simulink model "nms_3Dmodel_inv_wAnkleCPG"  (R2016b)
settings: Solver=ode3  StartTime=0.0  StopTime=tend  FixedStep=ts  RelTol=1e-3  EnableMultiTasking=on
InitFcn:
  | runScripts_inv;
values from neighbouring files (symbols this model uses):
  c = 0.05    [IID_nms_MechInit.m]    (also in nms_MechInit.m)
  c_jointstop = 0.3 / (pi/180)    (= 17.1887338539)    [IID_nms_MechInit.m]    (also in nms_MechInit.m)
  CPG_On = 1    [setCPGPar.m]    (also in setCPGPar_inv.m)
  CtrlPar_FP = [alpha0 alpha_cd alpha_cv]    [setCtrlPar.m]
  CtrlPar_FP_R = [R_hipR0 R_hipR_cd R_hipR_cv]    [setCtrlPar.m]
  CtrlPar_LL = l_clr    [setCtrlPar.m]
  CtrlPar_St = [StPreStim St_M1 St_M2 St_M3 St_M4 St_M5 St_M11]    [setCtrlPar.m]
  CtrlPar_St_R = [R_StPreStim R_St_M1 R_St_M3 R_St_M4]    [setCtrlPar.m]
  CtrlPar_Sw = [SwPreStim SwPhasePari SwPhaseParii SwCtrlPar_H SwCtrlPar_A      SwCtrlPar_Ki SwCtrlPar_Kii SwCtrlPar_Kiii SwCtrlPar_StP]    [setCtrlPar.m]
  CtrlPar_Sw_R = [R_SwPreStim R_Sw_M6]    [setCtrlPar.m]
  CtrlPar_theta0 = parBlCtrl(1)      *1*pi/180    [setCtrlPar.m]
  CtrlPar_Tr = [Tr_St_sup Tr_Sw]    [setCtrlPar.m]
  CtrlPar_Tr_R = [R_Tr_St_sup R_Tr_Sw]    [setCtrlPar.m]
  eref = 0.04    [IID_nms_MechInit.m]    (also in nms_MechInit.m)
  FmaxBFSH = 350    [nms_MechInit.m]
  FmaxGAS = 1500    [IID_nms_MechInit.m]    (also in nms_MechInit.m)
  FmaxGLU = 1500    [IID_nms_MechInit.m]    (also in nms_MechInit.m)
  FmaxHAB = 3000    [nms_MechInit.m]
  FmaxHAD = 4500    [nms_MechInit.m]
  FmaxHAM = 3000    [IID_nms_MechInit.m]    (also in nms_MechInit.m)
  FmaxHFL = 2000    [IID_nms_MechInit.m]    (also in nms_MechInit.m)
  FmaxRF = 1200    [nms_MechInit.m]
  FmaxSOL = 4000    [IID_nms_MechInit.m]    (also in nms_MechInit.m)
  FmaxTA = 800    [IID_nms_MechInit.m]    (also in nms_MechInit.m)
  FmaxVAS = 6000    [IID_nms_MechInit.m]    (also in nms_MechInit.m)
  init_a_tgt = 70*pi/180    (= 1.2217304764)    [setInitPar.m]
  init_a_tgtR = 90*pi/180    (= 1.57079632679)    [setInitPar.m]
  K = 5    [IID_nms_MechInit.m]    (also in nms_MechInit.m)
  leg_l = [D12_T D12_S]    [nms_MechInit.m]
  LongDelay = 0.020    (= 0.02)    [IID_setCtrlPar.m]    (also in nms_MechInit.m = 0.01)
  LongLoopDelay = 0.030    (= 0.03)    [nms_MechInit.m]
  loptBFSH = 0.12    [nms_MechInit.m]
  loptGAS = 0.05    [IID_nms_MechInit.m]    (also in nms_MechInit.m)
  loptGLU = 0.11    [IID_nms_MechInit.m]    (also in nms_MechInit.m)
  loptHAB = 0.09    [nms_MechInit.m]
  loptHAD = 0.10    (= 0.1)    [nms_MechInit.m]
  loptHAM = 0.10    (= 0.1)    [IID_nms_MechInit.m]    (also in nms_MechInit.m)
  loptHFL = 0.11    [IID_nms_MechInit.m]    (also in nms_MechInit.m)
  loptRF = 0.08    [nms_MechInit.m]
  loptSOL = 0.04    [IID_nms_MechInit.m]    (also in nms_MechInit.m)
  loptTA = 0.06    [IID_nms_MechInit.m]    (also in nms_MechInit.m)
  loptVAS = 0.08    [IID_nms_MechInit.m]    (also in nms_MechInit.m)
  lslackBFSH = 0.10    (= 0.1)    [nms_MechInit.m]
  lslackGAS = 0.40    (= 0.4)    [IID_nms_MechInit.m]    (also in nms_MechInit.m)
  lslackGLU = 0.13    [IID_nms_MechInit.m]    (also in nms_MechInit.m)
  lslackHAB = 0.07    [nms_MechInit.m]
  lslackHAD = 0.18    [nms_MechInit.m]
  lslackHAM = 0.31    [IID_nms_MechInit.m]    (also in nms_MechInit.m)
  lslackHFL = 0.10    (= 0.1)    [IID_nms_MechInit.m]    (also in nms_MechInit.m)
  lslackRF = 0.35    [nms_MechInit.m]
  lslackSOL = 0.26    [IID_nms_MechInit.m]    (also in nms_MechInit.m)
  lslackTA = 0.24    [IID_nms_MechInit.m]    (also in nms_MechInit.m)
  lslackVAS = 0.23    [IID_nms_MechInit.m]    (also in nms_MechInit.m)
  massBFSH = 2    [nms_MechInit.m]
  massGAS = 0.45    [IID_nms_MechInit.m]    (also in nms_MechInit.m)
  massGLU = 1.4    [IID_nms_MechInit.m]    (also in nms_MechInit.m)
  massHAB = 1.145    [nms_MechInit.m]
  massHAD = 1.91    [nms_MechInit.m]
  massHAM = 1.82    [IID_nms_MechInit.m]    (also in nms_MechInit.m)
  massHFL = 1.87    [IID_nms_MechInit.m]    (also in nms_MechInit.m)
  massRF = 1    [nms_MechInit.m]
  massSOL = 1.36    [IID_nms_MechInit.m]    (also in nms_MechInit.m)
  massTA = 0.29    [IID_nms_MechInit.m]    (also in nms_MechInit.m)
  massVAS = 2.91    [IID_nms_MechInit.m]    (also in nms_MechInit.m)
  MidDelay = 0.010    (= 0.01)    [IID_setCtrlPar.m]    (also in nms_MechInit.m = 0.005)
  N = 1.5    [IID_nms_MechInit.m]    (also in cmaes_parfor.m = size(x,1); nms_MechInit.m)
  phi12_LowLimit = 70*pi/180    (= 1.2217304764)    [IID_nms_MechInit.m]    (also in nms_MechInit.m)
  phi12_UpLimit = 130*pi/180    (= 2.26892802759)    [IID_nms_MechInit.m]    (also in nms_MechInit.m)
  phi23_UpLimit = 175*pi/180    (= 3.05432619099)    [IID_nms_MechInit.m]    (also in nms_MechInit.m)
  phi34_UpLimit = 230*pi/180    (= 4.01425727959)    [IID_nms_MechInit.m]    (also in nms_MechInit.m)
  phi34R_LowLimit = -15*pi/180    (= -0.261799387799)    [nms_MechInit.m]
  phi34R_UpLimit = 50*pi/180    (= 0.872664625997)    [nms_MechInit.m]
  phimaxGASa = 110*pi/180    (= 1.91986217719)    [IID_nms_MechInit.m]    (also in nms_MechInit.m = 1.74532925199)
  phimaxGASk = 140*pi/180    (= 2.44346095279)    [IID_nms_MechInit.m]    (also in nms_MechInit.m)
  phimaxRFk = 165*pi/180    (= 2.87979326579)    [nms_MechInit.m]
  phimaxSOL = 110*pi/180    (= 1.91986217719)    [IID_nms_MechInit.m]    (also in nms_MechInit.m = 1.74532925199)
  phimaxTA = 80*pi/180    (= 1.3962634016)    [IID_nms_MechInit.m]    (also in nms_MechInit.m)
  phimaxVAS = 165*pi/180    (= 2.87979326579)    [IID_nms_MechInit.m]    (also in nms_MechInit.m)
  phirefBFSH = 160*pi/180    (= 2.79252680319)    [nms_MechInit.m]
  phirefGASa = 80*pi/180    (= 1.3962634016)    [IID_nms_MechInit.m]    (also in nms_MechInit.m)
  phirefGASk = 165*pi/180    (= 2.87979326579)    [IID_nms_MechInit.m]    (also in nms_MechInit.m)
  phirefGLU = 150*pi/180    (= 2.61799387799)    [IID_nms_MechInit.m]    (also in nms_MechInit.m = 2.09439510239)
  phirefHAB = 10*pi/180    (= 0.174532925199)    [nms_MechInit.m]
  phirefHAD = 15*pi/180    (= 0.261799387799)    [nms_MechInit.m]
  phirefHAMh = 155*pi/180    (= 2.70526034059)    [IID_nms_MechInit.m]    (also in nms_MechInit.m = 2.61799387799)
  phirefHAMk = 180*pi/180    (= 3.14159265359)    [IID_nms_MechInit.m]    (also in nms_MechInit.m)
  phirefHFL = 180*pi/180    (= 3.14159265359)    [IID_nms_MechInit.m]    (also in nms_MechInit.m = 2.79252680319)
  phirefRFh = 170*pi/180    (= 2.96705972839)    [nms_MechInit.m]
  phirefRFk = 125*pi/180    (= 2.18166156499)    [nms_MechInit.m]
  phirefSOL = 80*pi/180    (= 1.3962634016)    [IID_nms_MechInit.m]    (also in nms_MechInit.m = 1.57079632679)
  phirefTA = 110*pi/180    (= 1.91986217719)    [IID_nms_MechInit.m]    (also in nms_MechInit.m)
  phirefVAS = 125*pi/180    (= 2.18166156499)    [IID_nms_MechInit.m]    (also in nms_MechInit.m = 2.09439510239)
  phiScaleGASa = acos(rGASamin/rGASamax)/(phiminGASa-phimaxGASa)    [nms_MechInit.m]
  phiScaleGASk = acos(rGASkmin/rGASkmax)/(phiminGASk-phimaxGASk)    [nms_MechInit.m]
  phiScaleRFk = acos(rRFkmin/rRFkmax)/(phiminRFk-phimaxRFk)    [nms_MechInit.m]
  phiScaleSOL = acos(rSOLmin/rSOLmax)/(phiminSOL-phimaxSOL)    [nms_MechInit.m]
  phiScaleTA = acos(rTAmin/rTAmax)/(phiminTA-phimaxTA)    [nms_MechInit.m]
  phiScaleVAS = acos(rVASmin/rVASmax)/(phiminVAS-phimaxVAS)    [nms_MechInit.m]
  rBFSH = 0.04    [nms_MechInit.m]
  rGASamax = 0.06    [nms_MechInit.m]
  rGASkmax = 0.05    [nms_MechInit.m]
  rGLU = 0.10    (= 0.1)    [IID_nms_MechInit.m]    (also in nms_MechInit.m = 0.08)
  rHAB = 0.06    [nms_MechInit.m]
  rHAD = 0.03    [nms_MechInit.m]
  rHAMh = 0.08    [IID_nms_MechInit.m]    (also in nms_MechInit.m)
  rHAMk = 0.05    [IID_nms_MechInit.m]    (also in nms_MechInit.m)
  rHFL = 0.10    (= 0.1)    [IID_nms_MechInit.m]    (also in nms_MechInit.m = 0.08)
  rhoBFSH = 0.7    [nms_MechInit.m]
  rhoGASa = 0.7    [IID_nms_MechInit.m]    (also in nms_MechInit.m)
  rhoGASk = 0.7    [IID_nms_MechInit.m]    (also in nms_MechInit.m)
  rhoGLU = 0.5    [IID_nms_MechInit.m]    (also in nms_MechInit.m)
  rhoHAB = 0.7    [nms_MechInit.m]
  rhoHAD = 1    [nms_MechInit.m]
  rhoHAMh = 0.7    [IID_nms_MechInit.m]    (also in nms_MechInit.m = 0.5)
  rhoHAMk = 0.7    [IID_nms_MechInit.m]    (also in nms_MechInit.m = 0.5)
  rhoHFL = 0.5    [IID_nms_MechInit.m]    (also in nms_MechInit.m)
  rhoRFh = 0.3    [nms_MechInit.m]
  rhoRFk = 0.5    [nms_MechInit.m]
  rhoSOL = 0.5    [IID_nms_MechInit.m]    (also in nms_MechInit.m)
  rhoTA = 0.7    [IID_nms_MechInit.m]    (also in nms_MechInit.m)
  ... (+55 more)
libraries: simulink_extras x30, nmc x30, simulink x22, NMCCPG_Library x13, powerlib_meascontrol x5
(part 12 of 12)

== system nms_3Dmodel_inv_wAnkleCPG/NMC Model/Neural Control Layer (Spinal Cord Control)/L Swing Phase (sagittal)/kneeii_damp and hold &kneeiii_leg stop &kneeiv_stance preparation ==
  note: Knee Phase i
  CtrlPar : Inport
  a_tgt : Inport  Port=2
  LceRF : Inport  Port=3
  LceHAM : Inport  Port=4
  VceHAM : Inport  Port=5
  VceVAS : Inport  Port=6
  VceBFSH : Inport  Port=7
  VceRF : Inport  Port=8
  LceHFL : Inport  Port=9
  LceGLU : Inport  Port=10
  LceVAS : Inport  Port=11
  Enable : EnablePort  StatesWhenEnabling=reset  ZeroCross=off
  Compare To Constant : simulink/Logic and Bit Operations/Compare To Constant  relop=<=  const=0  OutDataTypeStr=uint8  ZeroCross=off
  Constant1 : Constant  Value=0  OutDataTypeStr=boolean
  Constant2 : Constant  Value=0  OutDataTypeStr=boolean
  Constant3 : Constant  Value=0  OutDataTypeStr=boolean
  Constant4 : Constant
  Constant5 : Constant
  Demux1 : Demux  Outputs=5
  Divide1 : Product
  Divide2 : Product
  Logical Operator : Logic  Operator=NOT  AllPortsSameDT=off  OutDataTypeStr=boolean
  Logical Operator1 : Logic  AllPortsSameDT=off  OutDataTypeStr=boolean
  Relational Operator : RelationalOperator  Operator=<=  OutDataTypeStr=boolean  ZeroCross=off  RndMeth=Nearest
  Relational Operator1 : RelationalOperator  OutDataTypeStr=boolean  ZeroCross=off  RndMeth=Nearest
  S-R Flip-Flop : simulink_extras/Flip Flops/S-R Flip-Flop  initial_condition=0
  S-R Flip-Flop1 : simulink_extras/Flip Flops/S-R Flip-Flop  initial_condition=0
  S-R Flip-Flop2 : simulink_extras/Flip Flops/S-R Flip-Flop  initial_condition=0
  Sum1 : Sum  Inputs=+-|  SaturateOnIntegerOverflow=on  InputSameDT=on  OutDataTypeStr=Inherit: Same as first input
  Sum2 : Sum  Inputs=++|  SaturateOnIntegerOverflow=on  InputSameDT=on  OutDataTypeStr=Inherit: Same as first input
  Sum3 : Sum  Inputs=+-|  SaturateOnIntegerOverflow=on  InputSameDT=on  OutDataTypeStr=Inherit: Same as first input
  Sum4 : Sum  Inputs=+-|  SaturateOnIntegerOverflow=on  InputSameDT=on  OutDataTypeStr=Inherit: Same as first input
  Sum5 : Sum  Inputs=++|  SaturateOnIntegerOverflow=on  InputSameDT=on  OutDataTypeStr=Inherit: Same as first input
  Terminator : Terminator
  Terminator1 : Terminator
  Terminator2 : Terminator
  kneeii_damp and hold : Subsystem  TreatAsAtomicUnit=on
  kneeiii_leg stop : Subsystem  TreatAsAtomicUnit=on
  kneeiv_stance preparation : Subsystem  TreatAsAtomicUnit=on
  parSwKii : Selector  InputPortWidth=Sw_i  IndexOptions=Index vector (dialog)  Indices=parSwKii_i  OutputSizes=1
  parSwKiii : Selector  InputPortWidth=Sw_i  IndexOptions=Index vector (dialog)  Indices=parSwKiii_i  OutputSizes=1
  parSwKiv : Selector  InputPortWidth=Sw_i  IndexOptions=Index vector (dialog)  Indices=parSwKiv_i  OutputSizes=1
  parSwPhii : Selector  InputPortWidth=Sw_i  IndexOptions=Index vector (dialog)  Indices=parSwPhii_i  OutputSizes=1
  SRF_Sw_kii : Outport  OutputWhenDisabled=reset  InitialOutput=0
  SBFSH_Sw_kii : Outport  Port=2  OutputWhenDisabled=reset  InitialOutput=0
  SHAM_Sw_kiii : Outport  Port=3  OutputWhenDisabled=reset  InitialOutput=0
  SBFSH_Sw_kiii : Outport  Port=4  OutputWhenDisabled=reset  InitialOutput=0
  SGAS_Sw_kiii : Outport  Port=5  OutputWhenDisabled=reset  InitialOutput=0
  SHFL_Sw_kiv : Outport  Port=6  OutputWhenDisabled=reset  InitialOutput=0
  SGLU_Sw_kiv : Outport  Port=7  OutputWhenDisabled=reset  InitialOutput=0
  SVAS_Sw_kiv : Outport  Port=8  OutputWhenDisabled=reset  InitialOutput=0
  wires:
  VceVAS/1 -> kneeii_damp and hold/3(VceVAS)
  LceVAS/1 -> kneeiv_stance preparation/5(lceVAS)
  LceGLU/1 -> kneeiv_stance preparation/4(lceGLU)
  LceHFL/1 -> kneeiv_stance preparation/3(LceHFL)
  VceRF/1 -> kneeii_damp and hold/5(VceRF)
  VceBFSH/1 -> kneeii_damp and hold/4(VceBFSH)
  VceHAM/1 -> Compare To Constant/1
  Compare To Constant/1 -> Logical Operator1/2
  LceHAM/1 -> Relational Operator1/1, kneeiii_leg stop/3(LceHAM)  "LceHAM"
  Sum4/1 -> Relational Operator1/2  "lceOffHAM"
  Divide2/1 -> Sum4/2
  Constant5/1 -> Sum4/1
  Demux1/5 -> Divide2/2  "a2lopt_HAM"
  Sum1/1 -> Divide2/1
  Demux1/4 -> Sum1/2  "aRef_HAM"
  Sum2/1 -> Sum1/1  "a_thr"
  Demux1/3 -> Sum2/2  "a_del"
  Logical Operator/1 -> kneeii_damp and hold/Enable
  LceRF/1 -> kneeii_damp and hold/6(LceRF), Relational Operator/1
  Sum5/1 -> Relational Operator/2  "lceOffRF"
  Demux1/2 -> Divide1/2  "a2lopt_RF"
  a_tgt/1 -> kneeiv_stance preparation/2(a_tgt), kneeiii_leg stop/2(a_tgt), kneeii_damp and hold/2(a_tgt), Sum3/1, Sum2/1
  Divide1/1 -> Sum5/2
  Constant4/1 -> Sum5/1
  Sum3/1 -> Divide1/1
  Demux1/1 -> Sum3/2  "aRef_RF"
  parSwPhii/1 -> Demux1/1
  kneeiv_stance preparation/3(SVAS_Sw_kiv) -> SVAS_Sw_kiv/1
  kneeiv_stance preparation/2(SGLU_Sw_kiv) -> SGLU_Sw_kiv/1
  kneeiv_stance preparation/1(SHFL_Sw_kiv) -> SHFL_Sw_kiv/1
  kneeiii_leg stop/3(SGAS_Sw_kiii) -> SGAS_Sw_kiii/1
  kneeiii_leg stop/2(SKFL_Sw_kiii) -> SBFSH_Sw_kiii/1
  kneeiii_leg stop/1(SHAM_Sw_kiii) -> SHAM_Sw_kiii/1
  kneeii_damp and hold/2(SBFSH_Sw_kii) -> SBFSH_Sw_kii/1
  kneeii_damp and hold/1(SRF_Sw_kii) -> SRF_Sw_kii/1
  parSwKiv/1 -> kneeiv_stance preparation/1(CtrlPar)
  parSwKiii/1 -> kneeiii_leg stop/1(CtrlPar)
  S-R Flip-Flop2/1 -> kneeiv_stance preparation/Enable
  S-R Flip-Flop1/1 -> Logical Operator1/1, kneeiii_leg stop/Enable
  parSwKii/1 -> kneeii_damp and hold/1(CtrlPar)
  S-R Flip-Flop/1 -> Logical Operator/1
  CtrlPar/1 -> parSwPhii/1, parSwKiv/1, parSwKiii/1, parSwKii/1
  Logical Operator1/1 -> S-R Flip-Flop2/1
  S-R Flip-Flop2/2 -> Terminator2/1
  Constant3/1 -> S-R Flip-Flop2/2
  Relational Operator1/1 -> S-R Flip-Flop1/1
  S-R Flip-Flop1/2 -> Terminator1/1
  Constant2/1 -> S-R Flip-Flop1/2
  Relational Operator/1 -> S-R Flip-Flop/1
  S-R Flip-Flop/2 -> Terminator/1
  Constant1/1 -> S-R Flip-Flop/2

== system nms_3Dmodel_inv_wAnkleCPG/NMC Model/Neural Control Layer (Spinal Cord Control)/R Swing Phase (sagittal)/kneei_flexion from alpha ==
  note: Knee Phase i
  SBFSH : Inport
  Enable : EnablePort  StatesWhenEnabling=reset  ZeroCross=off
  SBFSH_Sw_ki : Outport  OutputWhenDisabled=reset  InitialOutput=0
  wires:
  SBFSH/1 -> SBFSH_Sw_ki/1

== system nms_3Dmodel_inv_wAnkleCPG/NMC Model/Neural Control Layer (Spinal Cord Control)/R Swing Phase (sagittal)/kneeii_damp and hold &kneeiii_leg stop &kneeiv_stance preparation ==
  note: Knee Phase i
  CtrlPar : Inport
  a_tgt : Inport  Port=2
  LceRF : Inport  Port=3
  LceHAM : Inport  Port=4
  VceHAM : Inport  Port=5
  VceVAS : Inport  Port=6
  VceBFSH : Inport  Port=7
  VceRF : Inport  Port=8
  LceHFL : Inport  Port=9
  LceGLU : Inport  Port=10
  LceVAS : Inport  Port=11
  Enable : EnablePort  StatesWhenEnabling=reset  ZeroCross=off
  Compare To Constant : simulink/Logic and Bit Operations/Compare To Constant  relop=<=  const=0  OutDataTypeStr=uint8  ZeroCross=off
  Constant1 : Constant  Value=0  OutDataTypeStr=boolean
  Constant2 : Constant  Value=0  OutDataTypeStr=boolean
  Constant3 : Constant  Value=0  OutDataTypeStr=boolean
  Constant4 : Constant
  Constant5 : Constant
  Demux1 : Demux  Outputs=5
  Divide1 : Product
  Divide2 : Product
  Logical Operator : Logic  Operator=NOT  AllPortsSameDT=off  OutDataTypeStr=boolean
  Logical Operator1 : Logic  AllPortsSameDT=off  OutDataTypeStr=boolean
  Relational Operator : RelationalOperator  Operator=<=  OutDataTypeStr=boolean  ZeroCross=off  RndMeth=Nearest
  Relational Operator1 : RelationalOperator  OutDataTypeStr=boolean  ZeroCross=off  RndMeth=Nearest
  S-R Flip-Flop : simulink_extras/Flip Flops/S-R Flip-Flop  initial_condition=0
  S-R Flip-Flop1 : simulink_extras/Flip Flops/S-R Flip-Flop  initial_condition=0
  S-R Flip-Flop2 : simulink_extras/Flip Flops/S-R Flip-Flop  initial_condition=0
  Sum1 : Sum  Inputs=+-|  SaturateOnIntegerOverflow=on  InputSameDT=on  OutDataTypeStr=Inherit: Same as first input
  Sum2 : Sum  Inputs=++|  SaturateOnIntegerOverflow=on  InputSameDT=on  OutDataTypeStr=Inherit: Same as first input
  Sum3 : Sum  Inputs=+-|  SaturateOnIntegerOverflow=on  InputSameDT=on  OutDataTypeStr=Inherit: Same as first input
  Sum4 : Sum  Inputs=+-|  SaturateOnIntegerOverflow=on  InputSameDT=on  OutDataTypeStr=Inherit: Same as first input
  Sum5 : Sum  Inputs=++|  SaturateOnIntegerOverflow=on  InputSameDT=on  OutDataTypeStr=Inherit: Same as first input
  Terminator : Terminator
  Terminator1 : Terminator
  Terminator2 : Terminator
  kneeii_damp and hold : Subsystem  TreatAsAtomicUnit=on
  kneeiii_leg stop : Subsystem  TreatAsAtomicUnit=on
  kneeiv_stance preparation : Subsystem  TreatAsAtomicUnit=on
  parSwKii : Selector  InputPortWidth=Sw_i  IndexOptions=Index vector (dialog)  Indices=parSwKii_i  OutputSizes=1
  parSwKiii : Selector  InputPortWidth=Sw_i  IndexOptions=Index vector (dialog)  Indices=parSwKiii_i  OutputSizes=1
  parSwKiv : Selector  InputPortWidth=Sw_i  IndexOptions=Index vector (dialog)  Indices=parSwKiv_i  OutputSizes=1
  parSwPhii : Selector  InputPortWidth=Sw_i  IndexOptions=Index vector (dialog)  Indices=parSwPhii_i  OutputSizes=1
  SRF_Sw_kii : Outport  OutputWhenDisabled=reset  InitialOutput=0
  SBFSH_Sw_kii : Outport  Port=2  OutputWhenDisabled=reset  InitialOutput=0
  SHAM_Sw_kiii : Outport  Port=3  OutputWhenDisabled=reset  InitialOutput=0
  SBFSH_Sw_kiii : Outport  Port=4  OutputWhenDisabled=reset  InitialOutput=0
  SGAS_Sw_kiii : Outport  Port=5  OutputWhenDisabled=reset  InitialOutput=0
  SHFL_Sw_kiv : Outport  Port=6  OutputWhenDisabled=reset  InitialOutput=0
  SGLU_Sw_kiv : Outport  Port=7  OutputWhenDisabled=reset  InitialOutput=0
  SVAS_Sw_kiv : Outport  Port=8  OutputWhenDisabled=reset  InitialOutput=0
  wires:
  VceVAS/1 -> kneeii_damp and hold/3(VceVAS)
  LceVAS/1 -> kneeiv_stance preparation/5(lceVAS)
  LceGLU/1 -> kneeiv_stance preparation/4(lceGLU)
  LceHFL/1 -> kneeiv_stance preparation/3(LceHFL)
  VceRF/1 -> kneeii_damp and hold/5(VceRF)
  VceBFSH/1 -> kneeii_damp and hold/4(VceBFSH)
  VceHAM/1 -> Compare To Constant/1
  Compare To Constant/1 -> Logical Operator1/2
  LceHAM/1 -> Relational Operator1/1, kneeiii_leg stop/3(LceHAM)  "LceHAM"
  Sum4/1 -> Relational Operator1/2  "lceOffHAM"
  Divide2/1 -> Sum4/2
  Constant5/1 -> Sum4/1
  Demux1/5 -> Divide2/2  "a2lopt_HAM"
  Sum1/1 -> Divide2/1
  Demux1/4 -> Sum1/2  "aRef_HAM"
  Sum2/1 -> Sum1/1  "a_thr"
  Demux1/3 -> Sum2/2  "a_del"
  Logical Operator/1 -> kneeii_damp and hold/Enable
  LceRF/1 -> Relational Operator/1, kneeii_damp and hold/6(LceRF)
  Sum5/1 -> Relational Operator/2  "lceOffRF"
  Demux1/2 -> Divide1/2  "a2lopt_RF"
  a_tgt/1 -> kneeiv_stance preparation/2(a_tgt), kneeiii_leg stop/2(a_tgt), kneeii_damp and hold/2(a_tgt), Sum3/1, Sum2/1
  Divide1/1 -> Sum5/2
  Constant4/1 -> Sum5/1
  Sum3/1 -> Divide1/1
  Demux1/1 -> Sum3/2  "aRef_RF"
  parSwPhii/1 -> Demux1/1
  kneeiv_stance preparation/3(SVAS_Sw_kiv) -> SVAS_Sw_kiv/1
  kneeiv_stance preparation/2(SGLU_Sw_kiv) -> SGLU_Sw_kiv/1
  kneeiv_stance preparation/1(SHFL_Sw_kiv) -> SHFL_Sw_kiv/1
  kneeiii_leg stop/3(SGAS_Sw_kiii) -> SGAS_Sw_kiii/1
  kneeiii_leg stop/2(SKFL_Sw_kiii) -> SBFSH_Sw_kiii/1
  kneeiii_leg stop/1(SHAM_Sw_kiii) -> SHAM_Sw_kiii/1
  kneeii_damp and hold/2(SBFSH_Sw_kii) -> SBFSH_Sw_kii/1
  kneeii_damp and hold/1(SRF_Sw_kii) -> SRF_Sw_kii/1
  parSwKiv/1 -> kneeiv_stance preparation/1(CtrlPar)
  parSwKiii/1 -> kneeiii_leg stop/1(CtrlPar)
  S-R Flip-Flop2/1 -> kneeiv_stance preparation/Enable
  S-R Flip-Flop1/1 -> Logical Operator1/1, kneeiii_leg stop/Enable
  parSwKii/1 -> kneeii_damp and hold/1(CtrlPar)
  S-R Flip-Flop/1 -> Logical Operator/1
  CtrlPar/1 -> parSwPhii/1, parSwKiv/1, parSwKiii/1, parSwKii/1
  Logical Operator1/1 -> S-R Flip-Flop2/1
  S-R Flip-Flop2/2 -> Terminator2/1
  Constant3/1 -> S-R Flip-Flop2/2
  Relational Operator1/1 -> S-R Flip-Flop1/1
  S-R Flip-Flop1/2 -> Terminator1/1
  Constant2/1 -> S-R Flip-Flop1/2
  Relational Operator/1 -> S-R Flip-Flop/1
  S-R Flip-Flop/2 -> Terminator/1
  Constant1/1 -> S-R Flip-Flop/2

== system nms_3Dmodel_inv_wAnkleCPG/NMC Model/CPG/CPG Output/Shape estimator left/Phase 1 ==
  Enable : EnablePort  StatesWhenEnabling=reset  ZeroCross=off
  Oscillator shape No Bias Inv : NMCCPG_Library/Oscillator shape No Bias Inv
  data_freq : DataStoreRead  DataStoreName=Freq_Ph1
  data_shape : DataStoreRead  DataStoreName=Shape_Ph1
  Shape_output : Outport  InitialOutput=0
  wires:
  Oscillator shape No Bias Inv/1 -> Shape_output/1
  data_freq/1 -> Oscillator shape No Bias Inv/2
  data_shape/1 -> Oscillator shape No Bias Inv/1

== system nms_3Dmodel_inv_wAnkleCPG/NMC Model/CPG/CPG Output/Shape estimator left/Phase 2 ==
  Enable : EnablePort  StatesWhenEnabling=reset  ZeroCross=off
  Oscillator shape No Bias Inv : NMCCPG_Library/Oscillator shape No Bias Inv
  data_freq : DataStoreRead  DataStoreName=Freq_Ph2
  data_shape : DataStoreRead  DataStoreName=Shape_Ph2
  Shape_output : Outport  InitialOutput=0
  wires:
  data_shape/1 -> Oscillator shape No Bias Inv/1
  data_freq/1 -> Oscillator shape No Bias Inv/2
  Oscillator shape No Bias Inv/1 -> Shape_output/1

== system nms_3Dmodel_inv_wAnkleCPG/NMC Model/CPG/CPG Output/Shape estimator left/Phase 3 ==
  Enable : EnablePort  StatesWhenEnabling=reset  ZeroCross=off
  Oscillator shape No Bias Inv : NMCCPG_Library/Oscillator shape No Bias Inv
  data_freq : DataStoreRead  DataStoreName=Freq_Ph3
  data_shape : DataStoreRead  DataStoreName=Shape_Ph3
  Shape_output : Outport  InitialOutput=0
  wires:
  Oscillator shape No Bias Inv/1 -> Shape_output/1
  data_freq/1 -> Oscillator shape No Bias Inv/2
  data_shape/1 -> Oscillator shape No Bias Inv/1

== system nms_3Dmodel_inv_wAnkleCPG/NMC Model/CPG/CPG Output/Shape estimator left/Phase 4 ==
  Enable : EnablePort  StatesWhenEnabling=reset  ZeroCross=off
  Oscillator shape No Bias Inv : NMCCPG_Library/Oscillator shape No Bias Inv
  data_freq : DataStoreRead  DataStoreName=Freq_Ph4
  data_shape : DataStoreRead  DataStoreName=Shape_Ph4
  Shape_output : Outport  InitialOutput=0
  wires:
  data_shape/1 -> Oscillator shape No Bias Inv/1
  data_freq/1 -> Oscillator shape No Bias Inv/2
  Oscillator shape No Bias Inv/1 -> Shape_output/1

== system nms_3Dmodel_inv_wAnkleCPG/NMC Model/CPG/Learning center/Phase 1/SaveToWorkspace ==
  Saver_shape : Inport
  Saver_freq : Inport  Port=2
  Enable : EnablePort
  data_store_freq : DataStoreWrite  DataStoreName=Freq_Ph1
  data_store_shape : DataStoreWrite  DataStoreName=Shape_Ph1
  wires:
  Saver_shape/1 -> data_store_shape/1
  Saver_freq/1 -> data_store_freq/1

== system nms_3Dmodel_inv_wAnkleCPG/NMC Model/CPG/Learning center/Phase 2/SaveToWorkspace ==
  Saver_shape : Inport
  Saver_freq : Inport  Port=2
  Enable : EnablePort
  data_store_freq : DataStoreWrite  DataStoreName=Freq_Ph2
  data_store_shape : DataStoreWrite  DataStoreName=Shape_Ph2
  wires:
  Saver_freq/1 -> data_store_freq/1
  Saver_shape/1 -> data_store_shape/1

== system nms_3Dmodel_inv_wAnkleCPG/NMC Model/CPG/Learning center/Phase 3/SaveToWorkspace ==
  Saver_shape : Inport
  Saver_freq : Inport  Port=2
  Enable : EnablePort
  data_store_freq : DataStoreWrite  DataStoreName=Freq_Ph3
  data_store_shape : DataStoreWrite  DataStoreName=Shape_Ph3
  wires:
  Saver_freq/1 -> data_store_freq/1
  Saver_shape/1 -> data_store_shape/1

== system nms_3Dmodel_inv_wAnkleCPG/NMC Model/CPG/Learning center/Phase 4/SaveToWorkspace ==
  Saver_shape : Inport
  Saver_freq : Inport  Port=2
  Enable : EnablePort
  data_store_freq : DataStoreWrite  DataStoreName=Freq_Ph4
  data_store_shape : DataStoreWrite  DataStoreName=Shape_Ph4
  wires:
  Saver_shape/1 -> data_store_shape/1
  Saver_freq/1 -> data_store_freq/1

== system nms_3Dmodel_inv_wAnkleCPG/NMC Model/Neural Control Layer (Spinal Cord Control)/L Swing Phase (sagittal)/kneeii_damp and hold &kneeiii_leg stop &kneeiv_stance preparation/kneeii_damp and hold ==
  note: Knee Phase i
  CtrlPar : Inport
  a_tgt : Inport  Port=2
  VceVAS : Inport  Port=3
  VceBFSH : Inport  Port=4
  VceRF : Inport  Port=5
  LceRF : Inport  Port=6
  Enable : EnablePort  StatesWhenEnabling=reset  ZeroCross=off
  Constant5 : Constant
  Demux2 : Demux  Outputs=5
  Divide1 : Product
  Divide2 : Product  Inputs=3
  Divide3 : Product  Inputs=*/
  Divide4 : Product  Inputs=*/
  Divide5 : Product
  Divide6 : Product
  Divide7 : Product  Inputs=*/
  Sum1 : Sum  Inputs=|-+  SaturateOnIntegerOverflow=on  InputSameDT=on  OutDataTypeStr=Inherit: Same as first input
  Sum10 : Sum  Inputs=|++  SaturateOnIntegerOverflow=on  InputSameDT=on  OutDataTypeStr=Inherit: Same as first input
  Sum2 : Sum  Inputs=|-+  SaturateOnIntegerOverflow=on  InputSameDT=on  OutDataTypeStr=Inherit: Same as first input
  Sum7 : Sum  Inputs=|++  SaturateOnIntegerOverflow=on  InputSameDT=on  OutDataTypeStr=Inherit: Same as first input
  positive half{,1..3} (4 alike) : Saturate  UpperLimit=inf  LowerLimit=0  ZeroCross=off
  SRF_Sw_kii : Outport  OutputWhenDisabled=reset  InitialOutput=0
  SBFSH_Sw_kii : Outport  Port=2  OutputWhenDisabled=reset  InitialOutput=0
  wires:
  Divide4/1 -> Sum7/2
  Divide3/1 -> Sum7/1
  VceVAS/1 -> positive half3/1
  Divide2/1 -> SBFSH_Sw_kii/1
  Divide7/1 -> positive half2/1
  Sum2/1 -> Divide7/1
  LceRF/1 -> Sum2/2
  Sum10/1 -> Sum2/1  "lceOffRF"
  Constant5/1 -> Sum10/2
  Divide6/1 -> Sum10/1
  Sum1/1 -> Divide6/2
  Demux2/5 -> Sum1/1  "aRef_RF"
  a_tgt/1 -> Sum1/2
  positive half2/1 -> Divide2/3
  Sum7/1 -> positive half1/1
  Demux2/4 -> Divide7/2, Divide6/1, Divide4/2  "a2lopt_RF"
  VceRF/1 -> Divide4/1
  Demux2/3 -> Divide3/2  "phi2lopt_BFSH"
  positive half1/1 -> Divide2/2
  Divide1/1 -> Divide2/1
  Demux2/2 -> Divide1/2  "VGainBFSH"
  positive half/1 -> Divide1/1
  positive half3/1 -> Divide5/1
  Divide5/1 -> SRF_Sw_kii/1
  VceBFSH/1 -> Divide3/1, positive half/1
  Demux2/1 -> Divide5/2  "VGainVAS_RF"
  CtrlPar/1 -> Demux2/1

== system nms_3Dmodel_inv_wAnkleCPG/NMC Model/Neural Control Layer (Spinal Cord Control)/L Swing Phase (sagittal)/kneeii_damp and hold &kneeiii_leg stop &kneeiv_stance preparation/kneeiii_leg stop ==
  note: Knee Phase iii
  CtrlPar : Inport
  a_tgt : Inport  Port=2
  LceHAM : Inport  Port=3
  Enable : EnablePort  StatesWhenEnabling=reset  ZeroCross=off
  Constant5 : Constant
  Demux1 : Demux  Outputs=7
  Divide{1..2,5,22} (4 alike) : Product
  Sum1 : Sum  Inputs=-+|  SaturateOnIntegerOverflow=on  InputSameDT=on  OutDataTypeStr=Inherit: Same as first input
  Sum10 : Sum  Inputs=+-|  SaturateOnIntegerOverflow=on  InputSameDT=on  OutDataTypeStr=Inherit: Same as first input
  Sum2 : Sum  Inputs=++|  SaturateOnIntegerOverflow=on  InputSameDT=on  OutDataTypeStr=Inherit: Same as first input
  Sum3 : Sum  Inputs=+-|  SaturateOnIntegerOverflow=on  InputSameDT=on  OutDataTypeStr=Inherit: Same as first input
  Sum4 : Sum  Inputs=+-|  SaturateOnIntegerOverflow=on  InputSameDT=on  OutDataTypeStr=Inherit: Same as first input
  positive half1 : Saturate  UpperLimit=inf  LowerLimit=0  ZeroCross=off
  positive half2 : Saturate  UpperLimit=inf  LowerLimit=0  ZeroCross=off
  SHAM_Sw_kiii : Outport  OutputWhenDisabled=reset  InitialOutput=0
  SKFL_Sw_kiii : Outport  Port=2  OutputWhenDisabled=reset  InitialOutput=0
  SGAS_Sw_kiii : Outport  Port=3  OutputWhenDisabled=reset  InitialOutput=0
  wires:
  Demux1/7 -> Divide2/2  "SGainHAM_GAS"
  Divide2/1 -> SGAS_Sw_kiii/1
  Divide1/1 -> SKFL_Sw_kiii/1
  Demux1/6 -> Divide1/2  "SGainHAM_KFL"
  positive half1/1 -> Divide2/1, Divide1/1
  Demux1/5 -> Sum4/2  "SHAM_thr"
  Sum4/1 -> positive half1/1
  Divide5/1 -> SHAM_Sw_kiii/1, Sum4/1  "S_HAM"
  Demux1/4 -> Divide5/2  "LGainHAM"
  Sum10/1 -> Sum1/1  "lceOffHAM"
  Demux1/3 -> Divide22/2  "a2lopt_HAM"
  Sum3/1 -> Divide22/1
  Demux1/2 -> Sum3/2  "aRef_HAM"
  Sum2/1 -> Sum3/1  "a_thr"
  Demux1/1 -> Sum2/2  "a_del"
  a_tgt/1 -> Sum2/1
  Divide22/1 -> Sum10/2
  Constant5/1 -> Sum10/1
  positive half2/1 -> Divide5/1  "del_lce"
  LceHAM/1 -> Sum1/2  "LceHAM"
  Sum1/1 -> positive half2/1  "del_LceMAN"
  CtrlPar/1 -> Demux1/1

== system nms_3Dmodel_inv_wAnkleCPG/NMC Model/Neural Control Layer (Spinal Cord Control)/L Swing Phase (sagittal)/kneeii_damp and hold &kneeiii_leg stop &kneeiv_stance preparation/kneeiv_stance preparation ==
  note: Knee Phase iii
  CtrlPar : Inport
  a_tgt : Inport  Port=2
  LceHFL : Inport  Port=3
  lceGLU : Inport  Port=4
  lceVAS : Inport  Port=5
  Enable : EnablePort  StatesWhenEnabling=reset  ZeroCross=off
  Constant1 : Constant
  Constant2 : Constant
  Constant5 : Constant  Value=pi/2
  Demux2 : Demux  Outputs=8
  Divide{1..3,5..6} (5 alike) : Product
  Sum1 : Sum  Inputs=-+|  SaturateOnIntegerOverflow=on  InputSameDT=on  OutDataTypeStr=Inherit: Same as first input
  Sum2 : Sum  Inputs=++|  SaturateOnIntegerOverflow=on  InputSameDT=on  OutDataTypeStr=Inherit: Same as first input
  Sum3 : Sum  Inputs=+-|  SaturateOnIntegerOverflow=on  InputSameDT=on  OutDataTypeStr=Inherit: Same as first input
  Sum4 : Sum  Inputs=+-|  SaturateOnIntegerOverflow=on  InputSameDT=on  OutDataTypeStr=Inherit: Same as first input
  Sum5 : Sum  Inputs=++|  SaturateOnIntegerOverflow=on  InputSameDT=on  OutDataTypeStr=Inherit: Same as first input
  Sum6 : Sum  Inputs=-+|  SaturateOnIntegerOverflow=on  InputSameDT=on  OutDataTypeStr=Inherit: Same as first input
  Sum7 : Sum  Inputs=+-|  SaturateOnIntegerOverflow=on  InputSameDT=on  OutDataTypeStr=Inherit: Same as first input
  Sum9 : Sum  Inputs=-+|  SaturateOnIntegerOverflow=on  InputSameDT=on  OutDataTypeStr=Inherit: Same as first input
  positive half1 : Saturate  UpperLimit=inf  LowerLimit=0  ZeroCross=off
  positive half2 : Saturate  UpperLimit=inf  LowerLimit=0  ZeroCross=off
  positive half3 : Saturate  UpperLimit=inf  LowerLimit=0  ZeroCross=off
  SHFL_Sw_kiv : Outport  OutputWhenDisabled=reset  InitialOutput=0
  SGLU_Sw_kiv : Outport  Port=2  OutputWhenDisabled=reset  InitialOutput=0
  SVAS_Sw_kiv : Outport  Port=3  OutputWhenDisabled=reset  InitialOutput=0
  wires:
  Demux2/8 -> Divide6/2  "LGainVAS"
  Demux2/7 -> Sum9/1  "loffVAS"
  Divide6/1 -> SVAS_Sw_kiv/1
  positive half3/1 -> Divide6/1
  lceVAS/1 -> Sum9/2
  Sum9/1 -> positive half3/1
  Sum7/1 -> Sum6/1  "lceOffGLU"
  Divide2/1 -> Sum7/2
  Constant2/1 -> Sum7/1
  Divide3/1 -> SGLU_Sw_kiv/1
  Demux2/6 -> Divide3/2  "LGainGLU"
  positive half1/1 -> Divide3/1
  lceGLU/1 -> Sum6/2  "lceGLU"
  Sum6/1 -> positive half1/1  "del_lce"
  Sum5/1 -> Sum1/1  "lceOffHFL"
  Divide1/1 -> Sum5/2
  Constant1/1 -> Sum5/1
  Divide5/1 -> SHFL_Sw_kiv/1
  Demux2/3 -> Divide5/2  "LGainHFL"
  Sum4/1 -> Divide2/1
  Demux2/4 -> Sum4/2  "phiRef_GLU"
  Demux2/5 -> Divide2/2  "phi2lopt_GLU"
  Demux2/2 -> Divide1/2  "phi2lopt_HFL"
  Sum3/1 -> Divide1/1
  Sum2/1 -> Sum4/1, Sum3/1
  Demux2/1 -> Sum3/2  "phiRef_HFL"
  Constant5/1 -> Sum2/1
  a_tgt/1 -> Sum2/2
  positive half2/1 -> Divide5/1
  LceHFL/1 -> Sum1/2
  Sum1/1 -> positive half2/1
  CtrlPar/1 -> Demux2/1

== system nms_3Dmodel_inv_wAnkleCPG/NMC Model/Neural Control Layer (Spinal Cord Control)/R Swing Phase (sagittal)/kneeii_damp and hold &kneeiii_leg stop &kneeiv_stance preparation/kneeii_damp and hold ==
  note: Knee Phase i
  CtrlPar : Inport
  a_tgt : Inport  Port=2
  VceVAS : Inport  Port=3
  VceBFSH : Inport  Port=4
  VceRF : Inport  Port=5
  LceRF : Inport  Port=6
  Enable : EnablePort  StatesWhenEnabling=reset  ZeroCross=off
  Constant5 : Constant
  Demux2 : Demux  Outputs=5
  Divide1 : Product
  Divide2 : Product  Inputs=3
  Divide3 : Product  Inputs=*/
  Divide4 : Product  Inputs=*/
  Divide5 : Product
  Divide6 : Product
  Divide7 : Product  Inputs=*/
  Sum1 : Sum  Inputs=|-+  SaturateOnIntegerOverflow=on  InputSameDT=on  OutDataTypeStr=Inherit: Same as first input
  Sum10 : Sum  Inputs=|++  SaturateOnIntegerOverflow=on  InputSameDT=on  OutDataTypeStr=Inherit: Same as first input
  Sum2 : Sum  Inputs=|-+  SaturateOnIntegerOverflow=on  InputSameDT=on  OutDataTypeStr=Inherit: Same as first input
  Sum7 : Sum  Inputs=|++  SaturateOnIntegerOverflow=on  InputSameDT=on  OutDataTypeStr=Inherit: Same as first input
  positive half{,1..3} (4 alike) : Saturate  UpperLimit=inf  LowerLimit=0  ZeroCross=off
  SRF_Sw_kii : Outport  OutputWhenDisabled=reset  InitialOutput=0
  SBFSH_Sw_kii : Outport  Port=2  OutputWhenDisabled=reset  InitialOutput=0
  wires:
  Divide4/1 -> Sum7/2
  Divide3/1 -> Sum7/1
  VceVAS/1 -> positive half3/1
  Divide2/1 -> SBFSH_Sw_kii/1
  Divide7/1 -> positive half2/1
  Sum2/1 -> Divide7/1
  LceRF/1 -> Sum2/2
  Sum10/1 -> Sum2/1  "lceOffRF"
  Constant5/1 -> Sum10/2
  Divide6/1 -> Sum10/1
  Sum1/1 -> Divide6/2
  Demux2/5 -> Sum1/1  "aRef_RF"
  a_tgt/1 -> Sum1/2
  positive half2/1 -> Divide2/3
  Sum7/1 -> positive half1/1
  Demux2/4 -> Divide7/2, Divide6/1, Divide4/2  "a2lopt_RF"
  VceRF/1 -> Divide4/1
  Demux2/3 -> Divide3/2  "phi2lopt_BFSH"
  positive half1/1 -> Divide2/2
  Divide1/1 -> Divide2/1
  Demux2/2 -> Divide1/2  "VGainBFSH"
  positive half/1 -> Divide1/1
  positive half3/1 -> Divide5/1
  Divide5/1 -> SRF_Sw_kii/1
  VceBFSH/1 -> Divide3/1, positive half/1
  Demux2/1 -> Divide5/2  "VGainVAS_RF"
  CtrlPar/1 -> Demux2/1

== system nms_3Dmodel_inv_wAnkleCPG/NMC Model/Neural Control Layer (Spinal Cord Control)/R Swing Phase (sagittal)/kneeii_damp and hold &kneeiii_leg stop &kneeiv_stance preparation/kneeiii_leg stop ==
  note: Knee Phase iii
  CtrlPar : Inport
  a_tgt : Inport  Port=2
  LceHAM : Inport  Port=3
  Enable : EnablePort  StatesWhenEnabling=reset  ZeroCross=off
  Constant5 : Constant
  Demux1 : Demux  Outputs=7
  Divide{1..2,5,22} (4 alike) : Product
  Sum1 : Sum  Inputs=-+|  SaturateOnIntegerOverflow=on  InputSameDT=on  OutDataTypeStr=Inherit: Same as first input
  Sum10 : Sum  Inputs=+-|  SaturateOnIntegerOverflow=on  InputSameDT=on  OutDataTypeStr=Inherit: Same as first input
  Sum2 : Sum  Inputs=++|  SaturateOnIntegerOverflow=on  InputSameDT=on  OutDataTypeStr=Inherit: Same as first input
  Sum3 : Sum  Inputs=+-|  SaturateOnIntegerOverflow=on  InputSameDT=on  OutDataTypeStr=Inherit: Same as first input
  Sum4 : Sum  Inputs=+-|  SaturateOnIntegerOverflow=on  InputSameDT=on  OutDataTypeStr=Inherit: Same as first input
  positive half1 : Saturate  UpperLimit=inf  LowerLimit=0  ZeroCross=off
  positive half2 : Saturate  UpperLimit=inf  LowerLimit=0  ZeroCross=off
  SHAM_Sw_kiii : Outport  OutputWhenDisabled=reset  InitialOutput=0
  SKFL_Sw_kiii : Outport  Port=2  OutputWhenDisabled=reset  InitialOutput=0
  SGAS_Sw_kiii : Outport  Port=3  OutputWhenDisabled=reset  InitialOutput=0
  wires:
  Demux1/7 -> Divide2/2  "SGainHAM_GAS"
  Divide2/1 -> SGAS_Sw_kiii/1
  Divide1/1 -> SKFL_Sw_kiii/1
  Demux1/6 -> Divide1/2  "SGainHAM_KFL"
  positive half1/1 -> Divide2/1, Divide1/1
  Demux1/5 -> Sum4/2  "SHAM_thr"
  Sum4/1 -> positive half1/1
  Divide5/1 -> SHAM_Sw_kiii/1, Sum4/1  "S_HAM"
  Demux1/4 -> Divide5/2  "LGainHAM"
  Sum10/1 -> Sum1/1  "lceOffHAM"
  Demux1/3 -> Divide22/2  "a2lopt_HAM"
  Sum3/1 -> Divide22/1
  Demux1/2 -> Sum3/2  "aRef_HAM"
  Sum2/1 -> Sum3/1  "a_thr"
  Demux1/1 -> Sum2/2  "a_del"
  a_tgt/1 -> Sum2/1
  Divide22/1 -> Sum10/2
  Constant5/1 -> Sum10/1
  positive half2/1 -> Divide5/1  "del_lce"
  LceHAM/1 -> Sum1/2  "LceHAM"
  Sum1/1 -> positive half2/1  "del_LceMAN"
  CtrlPar/1 -> Demux1/1

== system nms_3Dmodel_inv_wAnkleCPG/NMC Model/Neural Control Layer (Spinal Cord Control)/R Swing Phase (sagittal)/kneeii_damp and hold &kneeiii_leg stop &kneeiv_stance preparation/kneeiv_stance preparation ==
  note: Knee Phase iii
  CtrlPar : Inport
  a_tgt : Inport  Port=2
  LceHFL : Inport  Port=3
  lceGLU : Inport  Port=4
  lceVAS : Inport  Port=5
  Enable : EnablePort  StatesWhenEnabling=reset  ZeroCross=off
  Constant1 : Constant
  Constant2 : Constant
  Constant5 : Constant  Value=pi/2
  Demux2 : Demux  Outputs=8
  Divide{1..3,5..6} (5 alike) : Product
  Sum1 : Sum  Inputs=-+|  SaturateOnIntegerOverflow=on  InputSameDT=on  OutDataTypeStr=Inherit: Same as first input
  Sum2 : Sum  Inputs=++|  SaturateOnIntegerOverflow=on  InputSameDT=on  OutDataTypeStr=Inherit: Same as first input
  Sum3 : Sum  Inputs=+-|  SaturateOnIntegerOverflow=on  InputSameDT=on  OutDataTypeStr=Inherit: Same as first input
  Sum4 : Sum  Inputs=+-|  SaturateOnIntegerOverflow=on  InputSameDT=on  OutDataTypeStr=Inherit: Same as first input
  Sum5 : Sum  Inputs=++|  SaturateOnIntegerOverflow=on  InputSameDT=on  OutDataTypeStr=Inherit: Same as first input
  Sum6 : Sum  Inputs=-+|  SaturateOnIntegerOverflow=on  InputSameDT=on  OutDataTypeStr=Inherit: Same as first input
  Sum7 : Sum  Inputs=+-|  SaturateOnIntegerOverflow=on  InputSameDT=on  OutDataTypeStr=Inherit: Same as first input
  Sum9 : Sum  Inputs=-+|  SaturateOnIntegerOverflow=on  InputSameDT=on  OutDataTypeStr=Inherit: Same as first input
  positive half1 : Saturate  UpperLimit=inf  LowerLimit=0  ZeroCross=off
  positive half2 : Saturate  UpperLimit=inf  LowerLimit=0  ZeroCross=off
  positive half3 : Saturate  UpperLimit=inf  LowerLimit=0  ZeroCross=off
  SHFL_Sw_kiv : Outport  OutputWhenDisabled=reset  InitialOutput=0
  SGLU_Sw_kiv : Outport  Port=2  OutputWhenDisabled=reset  InitialOutput=0
  SVAS_Sw_kiv : Outport  Port=3  OutputWhenDisabled=reset  InitialOutput=0
  wires:
  Demux2/8 -> Divide6/2  "LGainVAS"
  Demux2/7 -> Sum9/1  "loffVAS"
  Divide6/1 -> SVAS_Sw_kiv/1
  positive half3/1 -> Divide6/1
  lceVAS/1 -> Sum9/2
  Sum9/1 -> positive half3/1
  Sum7/1 -> Sum6/1  "lceOffGLU"
  Divide2/1 -> Sum7/2
  Constant2/1 -> Sum7/1
  Divide3/1 -> SGLU_Sw_kiv/1
  Demux2/6 -> Divide3/2  "LGainGLU"
  positive half1/1 -> Divide3/1
  lceGLU/1 -> Sum6/2  "lceGLU"
  Sum6/1 -> positive half1/1  "del_lce"
  Sum5/1 -> Sum1/1  "lceOffHFL"
  Divide1/1 -> Sum5/2
  Constant1/1 -> Sum5/1
  Divide5/1 -> SHFL_Sw_kiv/1
  Demux2/3 -> Divide5/2  "LGainHFL"
  Sum4/1 -> Divide2/1
  Demux2/4 -> Sum4/2  "phiRef_GLU"
  Demux2/5 -> Divide2/2  "phi2lopt_GLU"
  Demux2/2 -> Divide1/2  "phi2lopt_HFL"
  Sum3/1 -> Divide1/1
  Sum2/1 -> Sum4/1, Sum3/1
  Demux2/1 -> Sum3/2  "phiRef_HFL"
  Constant5/1 -> Sum2/1
  a_tgt/1 -> Sum2/2
  positive half2/1 -> Divide5/1
  LceHFL/1 -> Sum1/2
  Sum1/1 -> positive half2/1
  CtrlPar/1 -> Demux2/1
